simulink model "DynamicKviMultiMicrogrid"  (R2022b)
settings: Solver=ode45  StartTime=0.0  StopTime=1000  RelTol=1e-3
values from neighbouring files (symbols this model uses):
  a_hidden_weights1 = zeros(n,h)    [Weights.m]
  a_hidden_weights2 = zeros(n,h)    [Weights.m]
  a_hidden_weights3 = zeros(n,h)    [Weights.m]
  a_input_weights1 = zeros(h,m)    [Weights.m]
  a_input_weights2 = zeros(h,m)    [Weights.m]
  a_input_weights3 = zeros(h,m)    [Weights.m]
  c_hidden_weights11 = zeros(100,1000)    [Training.m]
  c_hidden_weights12 = -1+(1+1)*rand(1,100,'single')    [Training.m]
  c_hidden_weights21 = zeros(100,1000)    [Training.m]
  c_hidden_weights22 = -1+(1+1)*rand(1,100,'single')    [Training.m]
  c_hidden_weights31 = zeros(100,1000)    [Training.m]
  c_hidden_weights32 = -1+(1+1)*rand(1,100,'single')    [Training.m]
  c_hidden_weights_a1 = -1+(1+1)*rand(1,100,'single')    [Training.m]
  c_hidden_weights_a2 = -1+(1+1)*rand(1,100,'single')    [Training.m]
  c_hidden_weights_a3 = -1+(1+1)*rand(1,100,'single')    [Training.m]
  c_input_weights1 = zeros(1000,m)    [Training.m]
  c_input_weights2 = zeros(1000,m)    [Training.m]
  c_input_weights3 = zeros(1000,m)    [Training.m]
  c_input_weights_a1 = zeros(100,n)    [Training.m]
  c_input_weights_a2 = zeros(100,n)    [Training.m]
  c_input_weights_a3 = zeros(100,n)    [Training.m]
libraries: simulink x9, slpidlib x3
settings Model: Creator=Vjatšeslav Škiparev  LastModifiedBy=assned
settings DataIOCC: LoggingIntervals=[0, 1000]
settings DebuggingCC: UnconnectedInputMsg=warning  UnconnectedOutputMsg=warning  UnconnectedLineMsg=warning
settings HardwareCC: ProdBitPerLong=64  ProdHWDeviceType=Intel->x86-64 (Linux 64)
settings ModelReferenceCC: EnableRefExpFcnMdlSchedulingChecks=on
settings RTWCC: DLArmComputeVersion=19.05

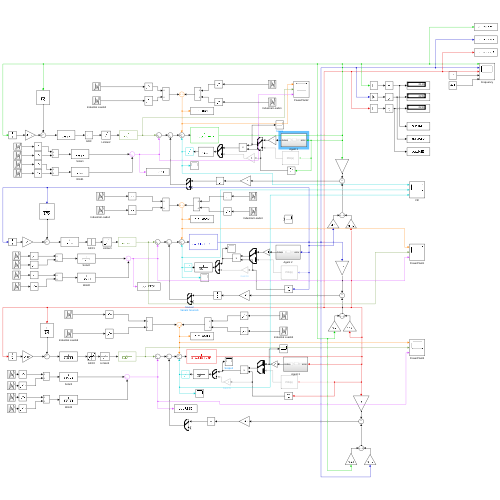
[thumbnail: Simulink's stored preview of the top-level diagram]
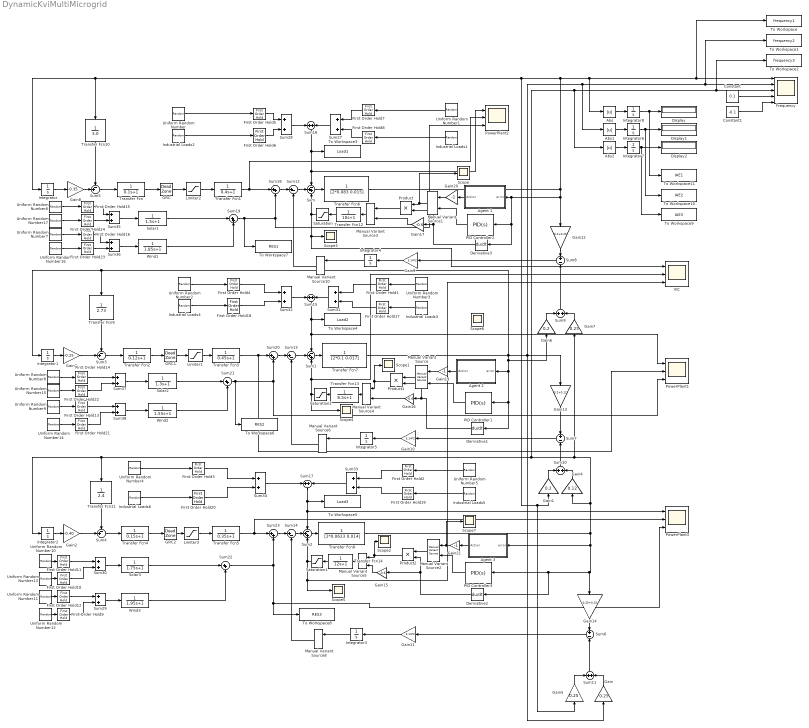
== system DynamicKviMultiMicrogrid ==
  Abs : Abs  SaturateOnIntegerOverflow=off
  Abs1 : Abs  SaturateOnIntegerOverflow=off
  Abs2 : Abs  SaturateOnIntegerOverflow=off
  Agent 1 : Subsystem
  Agent 2 : Subsystem
  Agent 3 : Subsystem
  Constant : Constant  Value=0.1
  Constant1 : Constant  Value=-0.1
  Derivative1 : Derivative
  Derivative2 : Derivative
  Derivative3 : Derivative
  Display : Display
  Display1 : Display
  Display2 : Display
  First Order Hold{1..24} (24 alike) : FirstOrderHold  ErrorTolerance=inf
  Frequency : Scope  NumInputPorts=5
  GRC : DeadZone  LowerValue=-0.12  UpperValue=0.12
  GRC1 : DeadZone  LowerValue=-0.12  UpperValue=0.12
  GRC2 : DeadZone  LowerValue=-0.12  UpperValue=0.12
  Gain : Gain  Gain=0.25
  Gain1 : Gain  Gain=0.2
  Gain10 : Gain  Gain=3.14*2
  Gain11 : Gain  Gain=3.14*2
  Gain12 : Gain  Gain=0.2+0.25
  Gain13 : Gain  Gain=0.2+0.12
  Gain14 : Gain  Gain=0.25+0.25
  Gain15 : Gain  Gain=-0.6
  Gain16 : Gain  Gain=-0.6
  Gain17 : Gain  Gain=-0.6
  Gain19 : Gain  Gain=-1
  Gain2 : Gain  Gain=-0.40
  Gain20 : Gain  Gain=-1
  Gain21 : Gain  Gain=-1
  Gain3 : Gain  Gain=-0.25
  Gain4 : Gain  Gain=0.12
  Gain5 : Gain  Gain=0.25
  Gain6 : Gain  Gain=0.2
  Gain7 : Gain  Gain=0.25
  Gain8 : Gain  Gain=-0.35
  Gain9 : Gain  Gain=3.14*2
  Industrial Loads1 : UniformRandomNumber  Minimum=-0.01  Maximum=0.01  SampleTime=1
  Industrial Loads2 : UniformRandomNumber  Minimum=-0.05  Maximum=0.05  SampleTime=2
  Industrial Loads3 : UniformRandomNumber  Minimum=-0.03  Maximum=0.03  SampleTime=5
  Industrial Loads4 : UniformRandomNumber  Minimum=-0.03  Maximum=0.03  SampleTime=5
  Industrial Loads5 : UniformRandomNumber  Minimum=-0.01  Maximum=0.01  SampleTime=2
  Industrial Loads6 : UniformRandomNumber  Minimum=-0.01  Maximum=0.01  SampleTime=2
  Integrator{,1..8} (9 alike) : Integrator
  Limiter1 : Saturate  UpperLimit=0.4  LowerLimit=0
  Limiter2 : Saturate  LowerLimit=0
  Limiter3 : Saturate  UpperLimit=0.3  LowerLimit=0
  Manual Variant Source{,1..6,8,10} (9 alike) : simulink/Signal Routing/Manual Variant Source  NumChoices=2  LabelModeActiveChoice=V_1
  PID Controller1 : slpidlib/PID Controller  Controller=PID  Form=Parallel  TimeDomain=Continuous-time  UseExternalTs=off  SampleTime=-1  IntegratorMethod=Forward Euler  FilterMethod=Forward Euler  ControllerParametersSource=internal  P=7.5  I=0.75  UseKiTs=off  D=0  N=100  UseFilter=on  TunerSelectOption=Transfer Function Based (PID Tuner App)  InitialConditionSource=internal  InitialConditionForIntegrator=0  InitialConditionForFilter=0  DifferentiatorICPrevScaledInput=0  ExternalReset=none  TrackingMode=off  Kt=1  LimitOutput=off  SatLimitsSource=internal  UpperSaturationLimit=inf  LowerSaturationLimit=-inf  LinearizeAsGain=on  AntiWindupMode=none  Kb=1  LimitIntegrator=off  UpperIntegratorSaturationLimit=inf  LowerIntegratorSaturationLimit=-inf  POutMin=[]  POutMax=[]  IOutMin=[]  IOutMax=[]  DOutMin=[]  DOutMax=[]  NOutMin=[]  NOutMax=[]  SumOutMin=[]  SumOutMax=[]  SaturationOutMin=[]  SaturationOutMax=[]  PParamMin=[]  PParamMax=[]  IParamMin=[]  IParamMax=[]  DParamMin=[]  DParamMax=[]  NParamMin=[]  NParamMax=[]  KbParamMin=[]  KbParamMax=[]  KtParamMin=[]  KtParamMax=[]  KbOutMin=[]  KbOutMax=[]  KtOutMin=[]  KtOutMax=[]  IntegratorOutMin=[]  IntegratorOutMax=[]  FilterOutMin=[]  FilterOutMax=[]  SumI1OutMin=[]  SumI1OutMax=[]  SumI2OutMin=[]  SumI2OutMax=[]  SumI3OutMin=[]  SumI3OutMax=[]  SumI4OutMin=[]  SumI4OutMax=[]  SumDOutMin=[]  SumDOutMax=[]  DifferentiatorOutMin=[]  DifferentiatorOutMax=[]  FilterDiffOutCoefMin=[]  FilterDiffOutCoefMax=[]  ReciprocalOutMin=[]  ReciprocalOutMax=[]  SumDenOutMin=[]  SumDenOutMax=[]  SumNumOutMin=[]  SumNumOutMax=[]  DivideOutMin=[]  DivideOutMax=[]  UdiffTsProdOutMin=[]  UdiffTsProdOutMax=[]  NTsProdOutMin=[]  NTsProdOutMax=[]  UintegralTsProdOutMin=[]  UintegralTsProdOutMax=[]  UngainTsProdOutMin=[]  UngainTsProdOutMax=[]  ClampingZeroOutDataTypeStr=Inherit: Inherit via back propagation  ClampingZeroOutMin=[]  ClampingZeroOutMax=[]  FilterDenConstantOutDataTypeStr=Inherit: Inherit via back propagation  FilterDenConstantOutMin=[]  FilterDenConstantOutMax=[]  PCopyOutDataTypeStr=Inherit: Inherit via back propagation  PCopyOutMin=[]  PCopyOutMax=[]  NCopyOutDataTypeStr=Inherit: Inherit via back propagation  NCopyOutMin=[]  NCopyOutMax=[]  IntegratorContinuousStateAttributes=''  IntegratorStateMustResolveToSignalObject=off  IntegratorRTWStateStorageClass=Auto  FilterContinuousStateAttributes=''  FilterStateMustResolveToSignalObject=off  FilterRTWStateStorageClass=Auto  ParallelPVariant=InternalParameters  IdealPVariant=Disabled  IVariant=InternalParameters  DVariant=InternalParameters  IntegratorVariant=Continuous  SatVariant=Disabled  AWVariant=Passthrough  PCopyVariant=Disabled  TRVariant=Disabled  FdbkBlocksVariant=Forward  IdealPFdbkVariant=Disabled  SatFdbkVariant=Disabled  DerivativeFilterVariant=ContFilter  NVariant=InternalParameters  NCopyVariant=Disabled  FilterICVariant=InternalICsFilter  IntegratorICVariant=InternalICs  ExternalResetVariant=Disabled  TRSumVariant=Passthrough  SumFdbkVariant=Disabled  SumVariant=Sum_PID  TsampFilterVariant=InternalTs  TsampNgainVariant=Passthrough  TsampIntegralVariant=Passthrough  ExternalSaturationOutDataTypeStr=Inherit: Same as second input
  PID Controller2 : slpidlib/PID Controller  Controller=PID  Form=Parallel  TimeDomain=Continuous-time  UseExternalTs=off  SampleTime=-1  IntegratorMethod=Forward Euler  FilterMethod=Forward Euler  ControllerParametersSource=internal  P=3.5  I=0.25  UseKiTs=off  D=0.5  N=100  UseFilter=on  TunerSelectOption=Transfer Function Based (PID Tuner App)  InitialConditionSource=internal  InitialConditionForIntegrator=0  InitialConditionForFilter=0  DifferentiatorICPrevScaledInput=0  ExternalReset=none  TrackingMode=off  Kt=1  LimitOutput=off  SatLimitsSource=internal  UpperSaturationLimit=inf  LowerSaturationLimit=-inf  LinearizeAsGain=on  AntiWindupMode=none  Kb=1  LimitIntegrator=off  UpperIntegratorSaturationLimit=inf  LowerIntegratorSaturationLimit=-inf  POutMin=[]  POutMax=[]  IOutMin=[]  IOutMax=[]  DOutMin=[]  DOutMax=[]  NOutMin=[]  NOutMax=[]  SumOutMin=[]  SumOutMax=[]  SaturationOutMin=[]  SaturationOutMax=[]  PParamMin=[]  PParamMax=[]  IParamMin=[]  IParamMax=[]  DParamMin=[]  DParamMax=[]  NParamMin=[]  NParamMax=[]  KbParamMin=[]  KbParamMax=[]  KtParamMin=[]  KtParamMax=[]  KbOutMin=[]  KbOutMax=[]  KtOutMin=[]  KtOutMax=[]  IntegratorOutMin=[]  IntegratorOutMax=[]  FilterOutMin=[]  FilterOutMax=[]  SumI1OutMin=[]  SumI1OutMax=[]  SumI2OutMin=[]  SumI2OutMax=[]  SumI3OutMin=[]  SumI3OutMax=[]  SumI4OutMin=[]  SumI4OutMax=[]  SumDOutMin=[]  SumDOutMax=[]  DifferentiatorOutMin=[]  DifferentiatorOutMax=[]  FilterDiffOutCoefMin=[]  FilterDiffOutCoefMax=[]  ReciprocalOutMin=[]  ReciprocalOutMax=[]  SumDenOutMin=[]  SumDenOutMax=[]  SumNumOutMin=[]  SumNumOutMax=[]  DivideOutMin=[]  DivideOutMax=[]  UdiffTsProdOutMin=[]  UdiffTsProdOutMax=[]  NTsProdOutMin=[]  NTsProdOutMax=[]  UintegralTsProdOutMin=[]  UintegralTsProdOutMax=[]  UngainTsProdOutMin=[]  UngainTsProdOutMax=[]  ClampingZeroOutDataTypeStr=Inherit: Inherit via back propagation  ClampingZeroOutMin=[]  ClampingZeroOutMax=[]  FilterDenConstantOutDataTypeStr=Inherit: Inherit via back propagation  FilterDenConstantOutMin=[]  FilterDenConstantOutMax=[]  PCopyOutDataTypeStr=Inherit: Inherit via back propagation  PCopyOutMin=[]  PCopyOutMax=[]  NCopyOutDataTypeStr=Inherit: Inherit via back propagation  NCopyOutMin=[]  NCopyOutMax=[]  IntegratorContinuousStateAttributes=''  IntegratorStateMustResolveToSignalObject=off  IntegratorRTWStateStorageClass=Auto  FilterContinuousStateAttributes=''  FilterStateMustResolveToSignalObject=off  FilterRTWStateStorageClass=Auto  ParallelPVariant=InternalParameters  IdealPVariant=Disabled  IVariant=InternalParameters  DVariant=InternalParameters  IntegratorVariant=Continuous  SatVariant=Disabled  AWVariant=Passthrough  PCopyVariant=Disabled  TRVariant=Disabled  FdbkBlocksVariant=Forward  IdealPFdbkVariant=Disabled  SatFdbkVariant=Disabled  DerivativeFilterVariant=ContFilter  NVariant=InternalParameters  NCopyVariant=Disabled  FilterICVariant=InternalICsFilter  IntegratorICVariant=InternalICs  ExternalResetVariant=Disabled  TRSumVariant=Passthrough  SumFdbkVariant=Disabled  SumVariant=Sum_PID  TsampFilterVariant=InternalTs  TsampNgainVariant=Passthrough  TsampIntegralVariant=Passthrough  ExternalSaturationOutDataTypeStr=Inherit: Same as second input
  PID Controller3 : slpidlib/PID Controller  Controller=PID  Form=Parallel  TimeDomain=Continuous-time  UseExternalTs=off  SampleTime=-1  IntegratorMethod=Forward Euler  FilterMethod=Forward Euler  ControllerParametersSource=internal  P=7.5  I=0.05  UseKiTs=off  D=0  N=100  UseFilter=on  TunerSelectOption=Transfer Function Based (PID Tuner App)  InitialConditionSource=internal  InitialConditionForIntegrator=0  InitialConditionForFilter=0  DifferentiatorICPrevScaledInput=0  ExternalReset=none  TrackingMode=off  Kt=1  LimitOutput=off  SatLimitsSource=internal  UpperSaturationLimit=inf  LowerSaturationLimit=-inf  LinearizeAsGain=on  AntiWindupMode=none  Kb=1  LimitIntegrator=off  UpperIntegratorSaturationLimit=inf  LowerIntegratorSaturationLimit=-inf  POutMin=[]  POutMax=[]  IOutMin=[]  IOutMax=[]  DOutMin=[]  DOutMax=[]  NOutMin=[]  NOutMax=[]  SumOutMin=[]  SumOutMax=[]  SaturationOutMin=[]  SaturationOutMax=[]  PParamMin=[]  PParamMax=[]  IParamMin=[]  IParamMax=[]  DParamMin=[]  DParamMax=[]  NParamMin=[]  NParamMax=[]  KbParamMin=[]  KbParamMax=[]  KtParamMin=[]  KtParamMax=[]  KbOutMin=[]  KbOutMax=[]  KtOutMin=[]  KtOutMax=[]  IntegratorOutMin=[]  IntegratorOutMax=[]  FilterOutMin=[]  FilterOutMax=[]  SumI1OutMin=[]  SumI1OutMax=[]  SumI2OutMin=[]  SumI2OutMax=[]  SumI3OutMin=[]  SumI3OutMax=[]  SumI4OutMin=[]  SumI4OutMax=[]  SumDOutMin=[]  SumDOutMax=[]  DifferentiatorOutMin=[]  DifferentiatorOutMax=[]  FilterDiffOutCoefMin=[]  FilterDiffOutCoefMax=[]  ReciprocalOutMin=[]  ReciprocalOutMax=[]  SumDenOutMin=[]  SumDenOutMax=[]  SumNumOutMin=[]  SumNumOutMax=[]  DivideOutMin=[]  DivideOutMax=[]  UdiffTsProdOutMin=[]  UdiffTsProdOutMax=[]  NTsProdOutMin=[]  NTsProdOutMax=[]  UintegralTsProdOutMin=[]  UintegralTsProdOutMax=[]  UngainTsProdOutMin=[]  UngainTsProdOutMax=[]  ClampingZeroOutDataTypeStr=Inherit: Inherit via back propagation  ClampingZeroOutMin=[]  ClampingZeroOutMax=[]  FilterDenConstantOutDataTypeStr=Inherit: Inherit via back propagation  FilterDenConstantOutMin=[]  FilterDenConstantOutMax=[]  PCopyOutDataTypeStr=Inherit: Inherit via back propagation  PCopyOutMin=[]  PCopyOutMax=[]  NCopyOutDataTypeStr=Inherit: Inherit via back propagation  NCopyOutMin=[]  NCopyOutMax=[]  IntegratorContinuousStateAttributes=''  IntegratorStateMustResolveToSignalObject=off  IntegratorRTWStateStorageClass=Auto  FilterContinuousStateAttributes=''  FilterStateMustResolveToSignalObject=off  FilterRTWStateStorageClass=Auto  ParallelPVariant=InternalParameters  IdealPVariant=Disabled  IVariant=InternalParameters  DVariant=InternalParameters  IntegratorVariant=Continuous  SatVariant=Disabled  AWVariant=Passthrough  PCopyVariant=Disabled  TRVariant=Disabled  FdbkBlocksVariant=Forward  IdealPFdbkVariant=Disabled  SatFdbkVariant=Disabled  DerivativeFilterVariant=ContFilter  NVariant=InternalParameters  NCopyVariant=Disabled  FilterICVariant=InternalICsFilter  IntegratorICVariant=InternalICs  ExternalResetVariant=Disabled  TRSumVariant=Passthrough  SumFdbkVariant=Disabled  SumVariant=Sum_PID  TsampFilterVariant=InternalTs  TsampNgainVariant=Passthrough  TsampIntegralVariant=Passthrough  ExternalSaturationOutDataTypeStr=Inherit: Same as second input
  PowerPlant1 : Scope  NumInputPorts=3
  PowerPlant2 : Scope  NumInputPorts=3
  PowerPlant3 : Scope  NumInputPorts=3
  Product : Product
  Product1 : Product
  Product2 : Product
  Saturation : Saturate  UpperLimit=0.25  LowerLimit=-0.25
  Saturation1 : Saturate  UpperLimit=0.1  LowerLimit=-0.1
  Saturation2 : Saturate  UpperLimit=0.25  LowerLimit=-0.25
  Scope{,1..7} (8 alike) : Scope
  Solar1 : TransferFcn  Denominator=[1.5 1]
  Solar2 : TransferFcn  Denominator=[1.3 1]
  Solar3 : TransferFcn  Denominator=[1.75 1]
  Sum : Sum  Inputs=-++
  Sum1 : Sum  Inputs=-++
  Sum{9..11,15..17,27..38} (18 alike) : Sum
  Sum12 : Sum  Inputs=|+-
  Sum13 : Sum  Inputs=|+-
  Sum14 : Sum  Inputs=|+-
  Sum{18..23} (6 alike) : Sum  Inputs=|++
  Sum2 : Sum  Inputs=-++
  Sum3 : Sum  Inputs=-+|
  Sum4 : Sum  Inputs=-+|
  Sum5 : Sum  Inputs=-+|
  Sum6 : Sum  Inputs=+-
  Sum7 : Sum  Inputs=+-
  Sum8 : Sum  Inputs=+-
  To Workspace : ToWorkspace  VariableName=frequency1  SampleTime=1
  To Workspace1 : ToWorkspace  VariableName=frequency2  SampleTime=1
  To Workspace10 : ToWorkspace  VariableName=IAE2  SampleTime=1
  To Workspace11 : ToWorkspace  VariableName=IAE1  SampleTime=1
  To Workspace2 : ToWorkspace  VariableName=frequency3  SampleTime=1
  To Workspace3 : ToWorkspace  VariableName=Load1  SampleTime=1
  To Workspace4 : ToWorkspace  VariableName=Load2  SampleTime=1
  To Workspace5 : ToWorkspace  VariableName=Load3  SampleTime=1
  To Workspace6 : ToWorkspace  VariableName=RES2  SampleTime=1
  To Workspace7 : ToWorkspace  VariableName=RES1  SampleTime=1
  To Workspace8 : ToWorkspace  VariableName=RES3  SampleTime=1
  To Workspace9 : ToWorkspace  VariableName=IAE3  SampleTime=1
  Transfer Fcn : TransferFcn  Denominator=[0.1 1]
  Transfer Fcn1 : TransferFcn  Denominator=[0.4 1]
  Transfer Fcn10 : TransferFcn  Denominator=[3.0]
  Transfer Fcn11 : TransferFcn  Denominator=[2.4]
  Transfer Fcn12 : TransferFcn  Denominator=[10 1]
  Transfer Fcn13 : TransferFcn  Denominator=[8.5 1]
  Transfer Fcn14 : TransferFcn  Denominator=[12 1]
  Transfer Fcn2 : TransferFcn  Denominator=[0.12 1]
  Transfer Fcn3 : TransferFcn  Denominator=[0.45 1]
  Transfer Fcn4 : TransferFcn  Denominator=[0.15 1]
  Transfer Fcn5 : TransferFcn  Denominator=[0.35 1]
  Transfer Fcn6 : TransferFcn  Denominator=[2*0.083 0.015]
  Transfer Fcn7 : TransferFcn  Denominator=[2*0.1 0.017]
  Transfer Fcn8 : TransferFcn  Denominator=[2*0.0623 0.014]
  Transfer Fcn9 : TransferFcn  Denominator=[2.73]
  Uniform Random Number : UniformRandomNumber  Minimum=0.15  Maximum=0.25  SampleTime=25
  Uniform Random Number1 : UniformRandomNumber  Minimum=0.35  Maximum=0.40  SampleTime=25
  Uniform Random Number10 : UniformRandomNumber  Minimum=0.05  Maximum=0.075  SampleTime=10
  Uniform Random Number11 : UniformRandomNumber  Minimum=0.05  Maximum=0.075  SampleTime=10
  Uniform Random Number12 : UniformRandomNumber  Minimum=-0.01  Maximum=0.01  SampleTime=1
  Uniform Random Number13 : UniformRandomNumber  Minimum=-0.05  Maximum=0.05  SampleTime=1
  Uniform Random Number14 : UniformRandomNumber  Minimum=-0.01  Maximum=0.01  SampleTime=1
  Uniform Random Number15 : UniformRandomNumber  Minimum=-0.01  Maximum=0.01  SampleTime=1
  Uniform Random Number16 : UniformRandomNumber  Minimum=-0.015  Maximum=0.015  SampleTime=2
  Uniform Random Number17 : UniformRandomNumber  Minimum=-0.015  Maximum=0.015  SampleTime=2
  Uniform Random Number2 : UniformRandomNumber  Minimum=0.2  Maximum=0.30  SampleTime=3
  Uniform Random Number3 : UniformRandomNumber  Minimum=0.225  Maximum=0.275  SampleTime=5
  Uniform Random Number4 : UniformRandomNumber  Minimum=0.15  Maximum=0.2  SampleTime=15
  Uniform Random Number5 : UniformRandomNumber  Minimum=0.075  Maximum=0.10  SampleTime=15
  Uniform Random Number6 : UniformRandomNumber  Minimum=0.10  Maximum=0.15  SampleTime=20
  Uniform Random Number7 : UniformRandomNumber  Minimum=0.10  Maximum=0.15  SampleTime=20
  Uniform Random Number8 : UniformRandomNumber  Minimum=0.125  Maximum=0.15  SampleTime=15
  Uniform Random Number9 : UniformRandomNumber  Minimum=0.05  Maximum=0.10  SampleTime=15
  VIC : Scope  NumInputPorts=3
  Wind1 : TransferFcn  Denominator=[1.85 1]
  Wind2 : TransferFcn  Denominator=[1.55 1]
  Wind3 : TransferFcn  Denominator=[1.95 1]
  wires:
  Sum1/1 -> Transfer Fcn7/1
  Sum2/1 -> Transfer Fcn8/1
  Sum/1 -> Transfer Fcn6/1
  Integrator/1 -> Gain8/1
  Sum5/1 -> Transfer Fcn/1
  Sum3/1 -> Transfer Fcn2/1
  Integrator1/1 -> Gain3/1
  Integrator2/1 -> Gain2/1
  Sum4/1 -> Transfer Fcn4/1
  Transfer Fcn9/1 -> Sum3/1
  Transfer Fcn10/1 -> Sum5/1
  Transfer Fcn11/1 -> Sum4/1
  Gain5/1 -> Sum11/1
  Gain/1 -> Sum11/2
  Gain4/1 -> Sum10/2
  Gain1/1 -> Sum10/1
  Gain3/1 -> Sum3/2
  Gain2/1 -> Sum4/2
  Gain6/1 -> Sum9/1
  Gain7/1 -> Sum9/2
  Gain8/1 -> Sum5/2
  Transfer Fcn14/1 -> Saturation1/1
  Saturation2/1 -> VIC/2, Sum1/3, Scope4/1
  Transfer Fcn12/1 -> Saturation/1
  Sum15/1 -> PowerPlant1/1, Sum1/1, To Workspace4/1
  Sum16/1 -> PowerPlant2/1, Sum/1, To Workspace3/1
  Sum17/1 -> To Workspace5/1, Sum2/1, PowerPlant3/1
  Uniform Random Number/1 -> First Order Hold5/1
  Uniform Random Number1/1 -> First Order Hold7/1
  Uniform Random Number2/1 -> First Order Hold4/1
  Uniform Random Number3/1 -> First Order Hold1/1
  Uniform Random Number4/1 -> First Order Hold3/1
  Uniform Random Number5/1 -> First Order Hold2/1
  Uniform Random Number6/1 -> First Order Hold15/1
  Uniform Random Number7/1 -> First Order Hold16/1
  Transfer Fcn1/1 -> Sum18/1, PowerPlant2/2
  Sum19/1 -> Sum18/2, PowerPlant2/3, To Workspace7/1
  Transfer Fcn3/1 -> PowerPlant1/2, Sum20/1
  Sum21/1 -> Sum20/2, PowerPlant1/3, To Workspace6/1
  Uniform Random Number8/1 -> First Order Hold14/1
  Uniform Random Number9/1 -> First Order Hold13/1
  Transfer Fcn5/1 -> PowerPlant3/2, Sum23/1
  Transfer Fcn13/1 -> Saturation2/1
  Saturation1/1 -> Sum2/3, Scope5/1, VIC/3
  Saturation/1 -> Sum/3, Scope3/1, VIC/1
  Wind3/1 -> Sum22/2
  Solar3/1 -> Sum22/1
  Solar2/1 -> Sum21/1
  Wind2/1 -> Sum21/2
  Wind1/1 -> Sum19/2
  Solar1/1 -> Sum19/1
  GRC/1 -> Limiter2/1
  Transfer Fcn/1 -> GRC/1
  Limiter2/1 -> Transfer Fcn1/1
  GRC1/1 -> Limiter1/1
  Transfer Fcn2/1 -> GRC1/1
  Limiter1/1 -> Transfer Fcn3/1
  GRC2/1 -> Limiter3/1
  Limiter3/1 -> Transfer Fcn5/1
  Transfer Fcn4/1 -> GRC2/1
  Sum18/1 -> Sum12/1
  Sum12/1 -> Sum/2
  Sum20/1 -> Sum13/1
  Sum13/1 -> Sum1/2
  Sum23/1 -> Sum14/1
  Sum14/1 -> Sum2/2
  Transfer Fcn6/1 -> Gain12/1, Derivative3/1, PID Controller2/1, Agent 1/1(error), Integrator/1, Transfer Fcn10/1, Gain1/1, Gain5/1, Abs/1, Frequency/1, To Workspace/1
  Sum8/1 -> Gain9/1
  Sum7/1 -> Gain10/1
  Sum6/1 -> Gain11/1
  First Order Hold7/1 -> Sum27/1
  Sum27/1 -> Sum16/2
  First Order Hold8/1 -> Sum27/2
  Industrial Loads1/1 -> First Order Hold8/1
  Sum28/1 -> Sum16/1
  First Order Hold5/1 -> Sum28/1
  First Order Hold6/1 -> Sum28/2
  Industrial Loads2/1 -> First Order Hold6/1
  First Order Hold9/1 -> Sum29/2
  Uniform Random Number12/1 -> First Order Hold9/1
  Uniform Random Number11/1 -> First Order Hold12/1
  Sum29/1 -> Wind3/1
  Uniform Random Number10/1 -> First Order Hold11/1
  Sum30/1 -> Solar3/1
  First Order Hold10/1 -> Sum30/2
  Uniform Random Number13/1 -> First Order Hold10/1
  First Order Hold11/1 -> Sum30/1
  First Order Hold12/1 -> Sum29/1
  First Order Hold17/1 -> Sum31/2
  Industrial Loads3/1 -> First Order Hold17/1
  First Order Hold1/1 -> Sum31/1
  Industrial Loads4/1 -> First Order Hold18/1
  First Order Hold18/1 -> Sum32/2
  First Order Hold4/1 -> Sum32/1
  Sum32/1 -> Sum15/1
  First Order Hold19/1 -> Sum33/2
  Industrial Loads5/1 -> First Order Hold19/1
  First Order Hold2/1 -> Sum33/1
  Sum33/1 -> Sum17/2
  First Order Hold20/1 -> Sum34/2
  Industrial Loads6/1 -> First Order Hold20/1
  Sum34/1 -> Sum17/1
  First Order Hold3/1 -> Sum34/1
  Manual Variant Source10/1 -> Sum12/2
  Manual Variant Source8/1 -> Sum14/2
  Manual Variant Source6/1 -> Sum13/2
  Gain9/1 -> Integrator4/1
  Gain10/1 -> Integrator5/1
  Gain11/1 -> Integrator3/1
  Gain12/1 -> Sum8/1
  Gain13/1 -> Sum7/1
  Gain14/1 -> Sum6/1
  PID Controller1/1 -> Manual Variant Source/2
  PID Controller3/1 -> Manual Variant Source2/2
  Sum35/1 -> Solar1/1
  First Order Hold15/1 -> Sum35/1
  Sum36/1 -> Wind1/1
  First Order Hold16/1 -> Sum36/1
  Sum37/1 -> Solar2/1
  Sum38/1 -> Wind2/1
  First Order Hold14/1 -> Sum37/1
  First Order Hold13/1 -> Sum38/1
  Uniform Random Number14/1 -> First Order Hold21/1
  First Order Hold21/1 -> Sum38/2
  Uniform Random Number15/1 -> First Order Hold22/1
  First Order Hold22/1 -> Sum37/2
  First Order Hold23/1 -> Sum36/2
  Uniform Random Number16/1 -> First Order Hold23/1
  Uniform Random Number17/1 -> First Order Hold24/1
  First Order Hold24/1 -> Sum35/2
  Integrator8/1 -> To Workspace11/1, Display/1
  Integrator6/1 -> To Workspace10/1, Display1/1
  Abs2/1 -> Integrator7/1
  Constant/1 -> Frequency/4
  Constant1/1 -> Frequency/5
  PID Controller2/1 -> Manual Variant Source1/2
  Manual Variant Source/1 -> Product1/1
  Manual Variant Source2/1 -> Product2/1
  Manual Variant Source4/1 -> Transfer Fcn13/1
  Manual Variant Source5/1 -> Transfer Fcn14/1
  Manual Variant Source3/1 -> Transfer Fcn12/1
  Gain16/1 -> Manual Variant Source4/2
  Gain17/1 -> Manual Variant Source3/2
  Derivative3/1 -> Gain17/1, Product/2
  Derivative1/1 -> Gain16/1, Product1/2
  Derivative2/1 -> Gain15/1, Product2/2
  Transfer Fcn7/1 -> Agent 2/1(error), PID Controller1/1, Derivative1/1, Gain6/1, Integrator1/1, Transfer Fcn9/1, Gain13/1, Gain/1, Abs1/1, To Workspace1/1, Frequency/2
  Product/1 -> Manual Variant Source3/1
  Product1/1 -> Scope1/1, Manual Variant Source4/1
  Product2/1 -> Scope2/1, Manual Variant Source5/1
  Gain15/1 -> Manual Variant Source5/2
  Sum9/1 -> Sum8/2
  Sum10/1 -> Sum7/2
  Sum11/1 -> Sum6/2
  Sum31/1 -> Sum15/2
  Abs/1 -> Integrator8/1
  Integrator7/1 -> Display2/1, To Workspace9/1
  Abs1/1 -> Integrator6/1
  Integrator5/1 -> Manual Variant Source6/1
  Integrator3/1 -> Manual Variant Source8/1
  Integrator4/1 -> Manual Variant Source10/1
  Transfer Fcn8/1 -> Integrator2/1, Transfer Fcn11/1, To Workspace2/1, Frequency/3, Abs2/1, Gain7/1, Gain4/1, Derivative2/1, PID Controller3/1, Gain14/1, Agent 3/1(error)
  Sum22/1 -> PowerPlant3/3, To Workspace8/1, Sum23/2
  Manual Variant Source1/1 -> Scope/1, Product/1
  Gain20/1 -> Manual Variant Source1/1
  Agent 1/1(Action) -> Gain20/1
  Gain19/1 -> Manual Variant Source/1
  Agent 2/1(Action) -> Gain19/1
  Gain21/1 -> Scope7/1, Manual Variant Source2/1
  Agent 3/1(Action) -> Gain21/1

== system DynamicKviMultiMicrogrid/Agent 1 ==
  error : Inport
  Gamma : Subsystem
  generate observations : Subsystem
  Action : Outport
  wires:
  error/1 -> Gamma/2(error), generate observations/1(error)
  generate observations/1(observations) -> Gamma/1(observations)
  Gamma/1(Action) -> Action/1

== system DynamicKviMultiMicrogrid/Agent 2 ==
  error : Inport
  Gamma : Subsystem
  generate observations : Subsystem
  Action : Outport
  wires:
  error/1 -> Gamma/2(error), generate observations/1(error)
  generate observations/1(observations) -> Gamma/1(observations)
  Gamma/1(Action) -> Action/1

== system DynamicKviMultiMicrogrid/Agent 3 ==
  error : Inport
  Gamma : Subsystem
  generate observations : Subsystem
  Action : Outport
  wires:
  error/1 -> Gamma/2(error), generate observations/1(error)
  generate observations/1(observations) -> Gamma/1(observations)
  Gamma/1(Action) -> Action/1

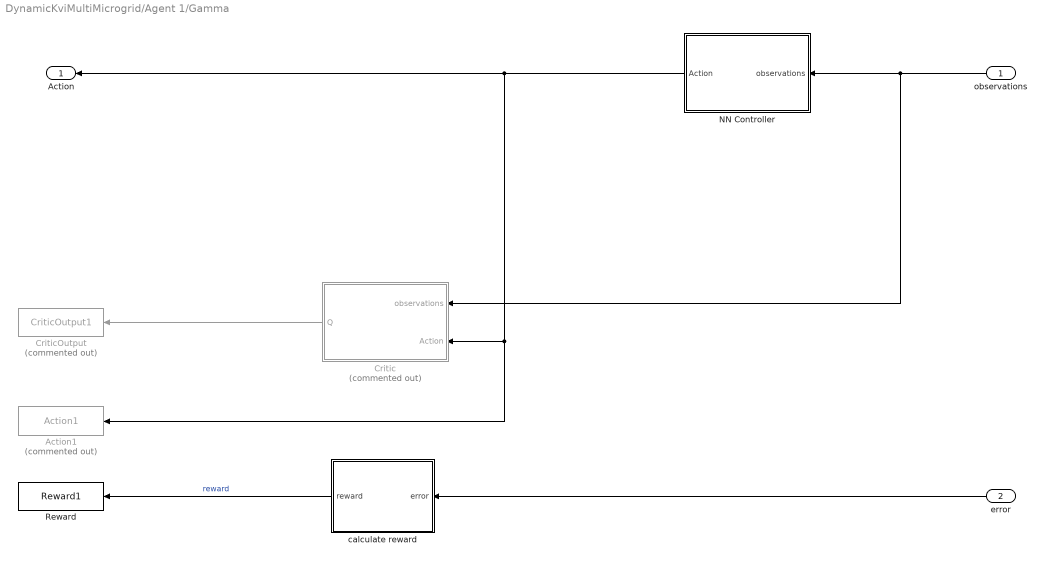
== system DynamicKviMultiMicrogrid/Agent 1/Gamma ==
  observations : Inport
  error : Inport  Port=2
  Action1 : ToWorkspace  Commented=on  VariableName=Action1  SampleTime=1
      settings: Save2DSignal=2-D array (concatenate along first dimension)
  Critic : Subsystem  Commented=on
  CriticOutput : ToWorkspace  Commented=on  VariableName=CriticOutput1  SampleTime=1
      settings: Save2DSignal=2-D array (concatenate along first dimension)
  NN Controller : Subsystem
  Reward : ToWorkspace  VariableName=Reward1  SampleTime=1
      settings: Save2DSignal=2-D array (concatenate along first dimension)
  calculate reward : Subsystem
  Action : Outport
  wires:
  NN Controller/1(Action) -> Action1/1, Critic/2(Action), Action/1
  observations/1 -> Critic/1(observations), NN Controller/1(observations)
  calculate reward/1(reward) -> Reward/1  "reward"
  Critic/1(Q) -> CriticOutput/1
  error/1 -> calculate reward/1(error)

== system DynamicKviMultiMicrogrid/Agent 1/generate observations ==
  error : Inport
  Derivative : Derivative
  Integrator : Integrator  IgnoreLimit=on
  Mux : Mux  Inputs=3
  observations : Outport  VectorParamsAs1DForOutWhenUnconnected=off
  wires:
  Mux/1 -> observations/1
  Integrator/1 -> Mux/2
  Derivative/1 -> Mux/3
  error/1 -> Derivative/1, Mux/1, Integrator/1

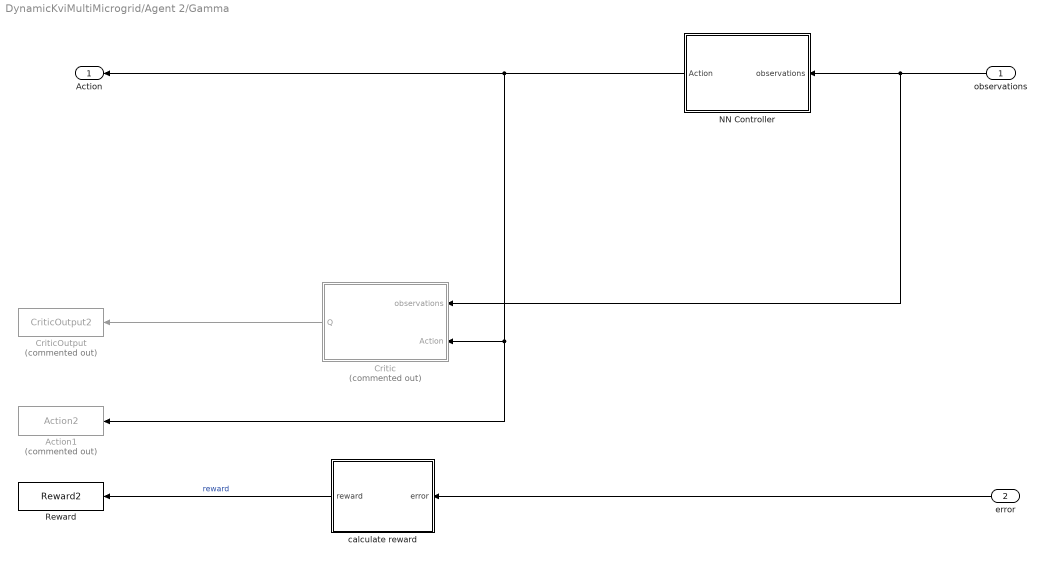
== system DynamicKviMultiMicrogrid/Agent 2/Gamma ==
  observations : Inport
  error : Inport  Port=2
  Action1 : ToWorkspace  Commented=on  VariableName=Action2  SampleTime=1
      settings: Save2DSignal=2-D array (concatenate along first dimension)
  Critic : Subsystem  Commented=on
  CriticOutput : ToWorkspace  Commented=on  VariableName=CriticOutput2  SampleTime=1
      settings: Save2DSignal=2-D array (concatenate along first dimension)
  NN Controller : Subsystem
  Reward : ToWorkspace  VariableName=Reward2  SampleTime=1
      settings: Save2DSignal=2-D array (concatenate along first dimension)
  calculate reward : Subsystem
  Action : Outport
  wires:
  NN Controller/1(Action) -> Action1/1, Critic/2(Action), Action/1
  observations/1 -> Critic/1(observations), NN Controller/1(observations)
  calculate reward/1(reward) -> Reward/1  "reward"
  Critic/1(Q) -> CriticOutput/1
  error/1 -> calculate reward/1(error)

== system DynamicKviMultiMicrogrid/Agent 2/generate observations ==
  error : Inport
  Derivative : Derivative
  Integrator : Integrator  IgnoreLimit=on
  Mux : Mux  Inputs=3
  observations : Outport  VectorParamsAs1DForOutWhenUnconnected=off
  wires:
  Mux/1 -> observations/1
  error/1 -> Derivative/1, Integrator/1, Mux/1
  Integrator/1 -> Mux/2
  Derivative/1 -> Mux/3

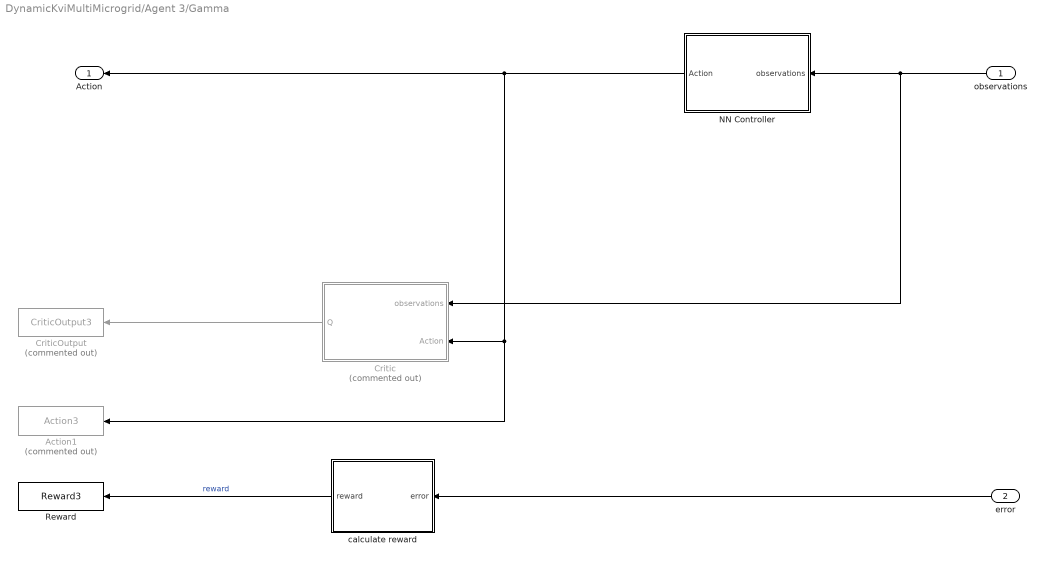
== system DynamicKviMultiMicrogrid/Agent 3/Gamma ==
  observations : Inport
  error : Inport  Port=2
  Action1 : ToWorkspace  Commented=on  VariableName=Action3  SampleTime=1
      settings: Save2DSignal=2-D array (concatenate along first dimension)
  Critic : Subsystem  Commented=on
  CriticOutput : ToWorkspace  Commented=on  VariableName=CriticOutput3  SampleTime=1
      settings: Save2DSignal=2-D array (concatenate along first dimension)
  NN Controller : Subsystem
  Reward : ToWorkspace  VariableName=Reward3  SampleTime=1
      settings: Save2DSignal=2-D array (concatenate along first dimension)
  calculate reward : Subsystem
  Action : Outport
  wires:
  NN Controller/1(Action) -> Action1/1, Critic/2(Action), Action/1
  observations/1 -> Critic/1(observations), NN Controller/1(observations)
  calculate reward/1(reward) -> Reward/1  "reward"
  Critic/1(Q) -> CriticOutput/1
  error/1 -> calculate reward/1(error)

== system DynamicKviMultiMicrogrid/Agent 3/generate observations ==
  error : Inport
  Derivative : Derivative
  Integrator : Integrator  IgnoreLimit=on
  Mux : Mux  Inputs=3
  observations : Outport  VectorParamsAs1DForOutWhenUnconnected=off
  wires:
  Mux/1 -> observations/1
  error/1 -> Derivative/1, Integrator/1, Mux/1
  Integrator/1 -> Mux/2
  Derivative/1 -> Mux/3

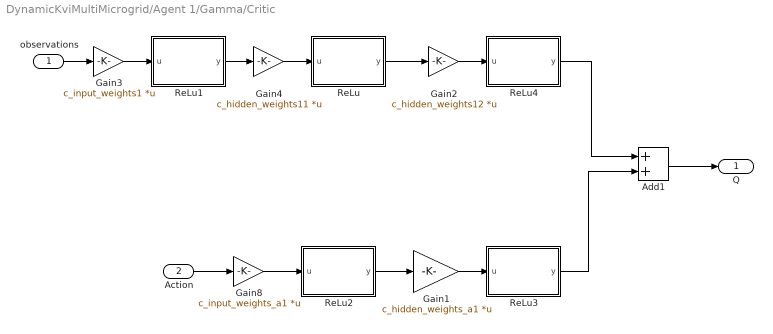
== system DynamicKviMultiMicrogrid/Agent 1/Gamma/Critic ==
  observations : Inport
  Action : Inport  Port=2
  Add1 : Sum
  Gain1 : Gain  Gain=c_hidden_weights_a1  Multiplication=Matrix(K*u)
  Gain2 : Gain  Gain=c_hidden_weights12  Multiplication=Matrix(K*u)
  Gain3 : Gain  Gain=c_input_weights1  Multiplication=Matrix(K*u)
  Gain4 : Gain  Gain=c_hidden_weights11  Multiplication=Matrix(K*u)
  Gain8 : Gain  Gain=c_input_weights_a1  Multiplication=Matrix(K*u)
  ReLu : MATLAB Function  TreatAsAtomicUnit=on
  ReLu1 : MATLAB Function  TreatAsAtomicUnit=on
  ReLu2 : MATLAB Function  TreatAsAtomicUnit=on
  ReLu3 : MATLAB Function  TreatAsAtomicUnit=on
  ReLu4 : MATLAB Function  TreatAsAtomicUnit=on
  Q : Outport
  wires:
  observations/1 -> Gain3/1
  Add1/1 -> Q/1
  Action/1 -> Gain8/1
  ReLu3/1(y) -> Add1/2
  Gain8/1 -> ReLu2/1(u)
  ReLu2/1(y) -> Gain1/1
  Gain1/1 -> ReLu3/1(u)
  Gain3/1 -> ReLu1/1(u)
  ReLu1/1(y) -> Gain4/1
  Gain4/1 -> ReLu/1(u)
  ReLu/1(y) -> Gain2/1
  Gain2/1 -> ReLu4/1(u)
  ReLu4/1(y) -> Add1/1

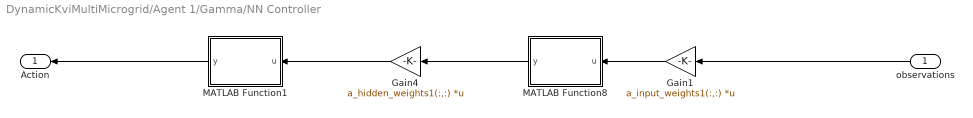
== system DynamicKviMultiMicrogrid/Agent 1/Gamma/NN Controller ==
  observations : Inport
  Gain1 : Gain  Gain=a_input_weights1(:,:)  Multiplication=Matrix(K*u)
  Gain4 : Gain  Gain=a_hidden_weights1(:,:)  Multiplication=Matrix(K*u)
  MATLAB Function1 : MATLAB Function  TreatAsAtomicUnit=on
  MATLAB Function8 : MATLAB Function  TreatAsAtomicUnit=on
  Action : Outport
  wires:
  Gain1/1 -> MATLAB Function8/1(u)
  Gain4/1 -> MATLAB Function1/1(u)
  MATLAB Function8/1(y) -> Gain4/1
  observations/1 -> Gain1/1
  MATLAB Function1/1(y) -> Action/1

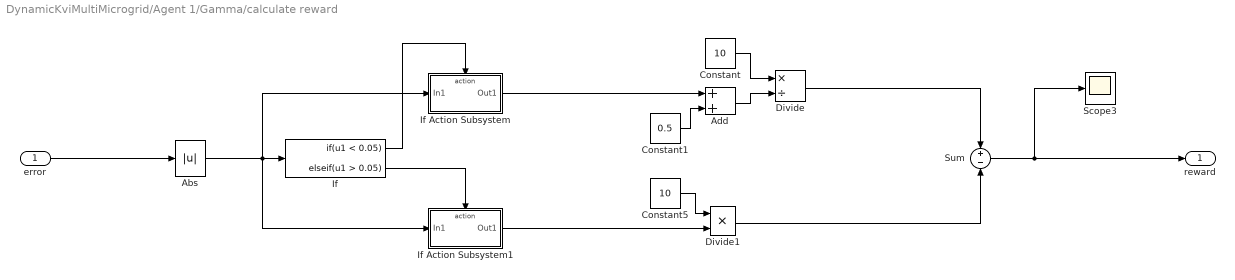
== system DynamicKviMultiMicrogrid/Agent 1/Gamma/calculate reward ==
  error : Inport
  Abs : Abs  SaturateOnIntegerOverflow=off
  Add : Sum
  Constant : Constant  Value=10
  Constant1 : Constant  Value=0.5  VectorParams1D=off
  Constant5 : Constant  Value=10  VectorParams1D=off
  Divide : Product  Inputs=*/
  Divide1 : Product  Inputs=**
  If : If  IfExpression=u1 < 0.05  ElseIfExpressions=u1 > 0.05  ShowElse=off
  If Action Subsystem : Subsystem  TreatAsAtomicUnit=on
  If Action Subsystem1 : Subsystem  TreatAsAtomicUnit=on
  Scope3 : Scope
  Sum : Sum  Inputs=+-  OutDataTypeStr=double
  reward : Outport  VectorParamsAs1DForOutWhenUnconnected=off
  wires:
  Constant/1 -> Divide/1
  Add/1 -> Divide/2
  Constant1/1 -> Add/2
  error/1 -> Abs/1
  Constant5/1 -> Divide1/1
  If Action Subsystem1/1(Out1) -> Divide1/2
  Divide/1 -> Sum/1
  If Action Subsystem/1(Out1) -> Add/1
  Sum/1 -> Scope3/1, reward/1
  If/2 -> If Action Subsystem1/Action
  If/1 -> If Action Subsystem/Action
  Abs/1 -> If/1, If Action Subsystem1/1(In1), If Action Subsystem/1(In1)
  Divide1/1 -> Sum/2

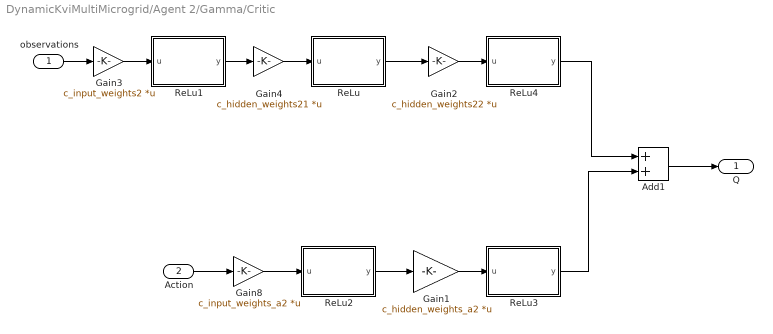
== system DynamicKviMultiMicrogrid/Agent 2/Gamma/Critic ==
  observations : Inport
  Action : Inport  Port=2
  Add1 : Sum
  Gain1 : Gain  Gain=c_hidden_weights_a2  Multiplication=Matrix(K*u)
  Gain2 : Gain  Gain=c_hidden_weights22  Multiplication=Matrix(K*u)
  Gain3 : Gain  Gain=c_input_weights2  Multiplication=Matrix(K*u)
  Gain4 : Gain  Gain=c_hidden_weights21  Multiplication=Matrix(K*u)
  Gain8 : Gain  Gain=c_input_weights_a2  Multiplication=Matrix(K*u)
  ReLu : MATLAB Function  TreatAsAtomicUnit=on
  ReLu1 : MATLAB Function  TreatAsAtomicUnit=on
  ReLu2 : MATLAB Function  TreatAsAtomicUnit=on
  ReLu3 : MATLAB Function  TreatAsAtomicUnit=on
  ReLu4 : MATLAB Function  TreatAsAtomicUnit=on
  Q : Outport
  wires:
  observations/1 -> Gain3/1
  Add1/1 -> Q/1
  Action/1 -> Gain8/1
  ReLu3/1(y) -> Add1/2
  Gain8/1 -> ReLu2/1(u)
  ReLu2/1(y) -> Gain1/1
  Gain1/1 -> ReLu3/1(u)
  Gain3/1 -> ReLu1/1(u)
  ReLu1/1(y) -> Gain4/1
  Gain4/1 -> ReLu/1(u)
  ReLu/1(y) -> Gain2/1
  Gain2/1 -> ReLu4/1(u)
  ReLu4/1(y) -> Add1/1

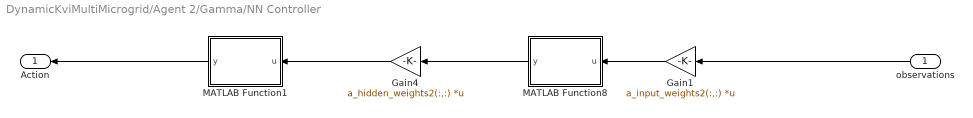
== system DynamicKviMultiMicrogrid/Agent 2/Gamma/NN Controller ==
  observations : Inport
  Gain1 : Gain  Gain=a_input_weights2(:,:)  Multiplication=Matrix(K*u)
  Gain4 : Gain  Gain=a_hidden_weights2(:,:)  Multiplication=Matrix(K*u)
  MATLAB Function1 : MATLAB Function  TreatAsAtomicUnit=on
  MATLAB Function8 : MATLAB Function  TreatAsAtomicUnit=on
  Action : Outport
  wires:
  Gain1/1 -> MATLAB Function8/1(u)
  Gain4/1 -> MATLAB Function1/1(u)
  MATLAB Function8/1(y) -> Gain4/1
  observations/1 -> Gain1/1
  MATLAB Function1/1(y) -> Action/1

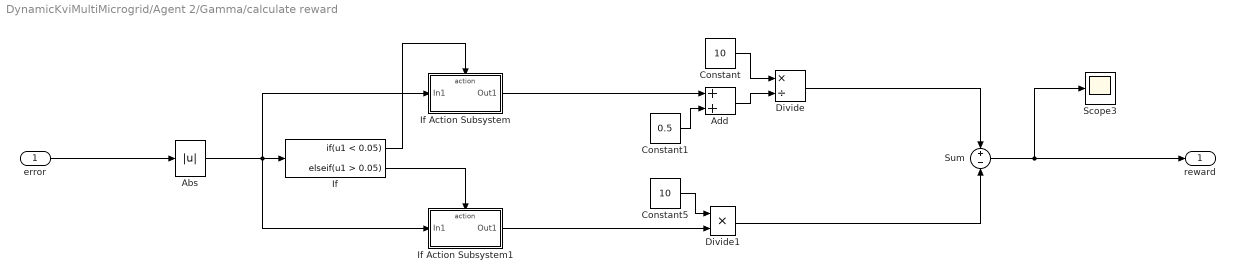
== system DynamicKviMultiMicrogrid/Agent 2/Gamma/calculate reward ==
  error : Inport
  Abs : Abs  SaturateOnIntegerOverflow=off
  Add : Sum
  Constant : Constant  Value=10
  Constant1 : Constant  Value=0.5  VectorParams1D=off
  Constant5 : Constant  Value=10  VectorParams1D=off
  Divide : Product  Inputs=*/
  Divide1 : Product  Inputs=**
  If : If  IfExpression=u1 < 0.05  ElseIfExpressions=u1 > 0.05  ShowElse=off
  If Action Subsystem : Subsystem  TreatAsAtomicUnit=on
  If Action Subsystem1 : Subsystem  TreatAsAtomicUnit=on
  Scope3 : Scope
  Sum : Sum  Inputs=+-  OutDataTypeStr=double
  reward : Outport  VectorParamsAs1DForOutWhenUnconnected=off
  wires:
  Constant/1 -> Divide/1
  Add/1 -> Divide/2
  Constant1/1 -> Add/2
  error/1 -> Abs/1
  Constant5/1 -> Divide1/1
  If Action Subsystem1/1(Out1) -> Divide1/2
  Divide/1 -> Sum/1
  If Action Subsystem/1(Out1) -> Add/1
  Sum/1 -> Scope3/1, reward/1
  If/2 -> If Action Subsystem1/Action
  If/1 -> If Action Subsystem/Action
  Abs/1 -> If/1, If Action Subsystem1/1(In1), If Action Subsystem/1(In1)
  Divide1/1 -> Sum/2

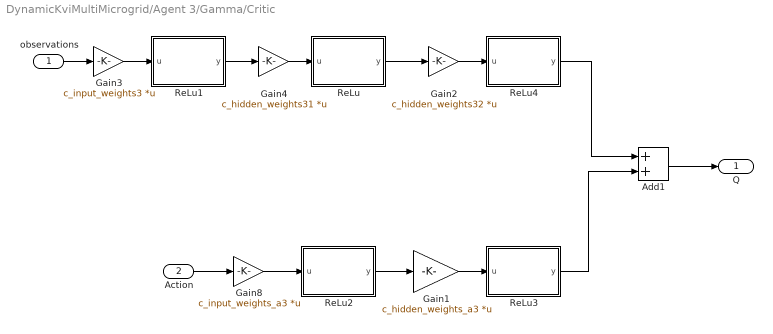
== system DynamicKviMultiMicrogrid/Agent 3/Gamma/Critic ==
  observations : Inport
  Action : Inport  Port=2
  Add1 : Sum
  Gain1 : Gain  Gain=c_hidden_weights_a3  Multiplication=Matrix(K*u)
  Gain2 : Gain  Gain=c_hidden_weights32  Multiplication=Matrix(K*u)
  Gain3 : Gain  Gain=c_input_weights3  Multiplication=Matrix(K*u)
  Gain4 : Gain  Gain=c_hidden_weights31  Multiplication=Matrix(K*u)
  Gain8 : Gain  Gain=c_input_weights_a3  Multiplication=Matrix(K*u)
  ReLu : MATLAB Function  TreatAsAtomicUnit=on
  ReLu1 : MATLAB Function  TreatAsAtomicUnit=on
  ReLu2 : MATLAB Function  TreatAsAtomicUnit=on
  ReLu3 : MATLAB Function  TreatAsAtomicUnit=on
  ReLu4 : MATLAB Function  TreatAsAtomicUnit=on
  Q : Outport
  wires:
  observations/1 -> Gain3/1
  Add1/1 -> Q/1
  Action/1 -> Gain8/1
  ReLu3/1(y) -> Add1/2
  Gain8/1 -> ReLu2/1(u)
  ReLu2/1(y) -> Gain1/1
  Gain1/1 -> ReLu3/1(u)
  Gain3/1 -> ReLu1/1(u)
  ReLu1/1(y) -> Gain4/1
  Gain4/1 -> ReLu/1(u)
  ReLu/1(y) -> Gain2/1
  Gain2/1 -> ReLu4/1(u)
  ReLu4/1(y) -> Add1/1

== system DynamicKviMultiMicrogrid/Agent 3/Gamma/NN Controller ==
  observations : Inport
  Gain1 : Gain  Gain=a_input_weights3(:,:)  Multiplication=Matrix(K*u)
  Gain4 : Gain  Gain=a_hidden_weights3(:,:)  Multiplication=Matrix(K*u)
  MATLAB Function1 : MATLAB Function  TreatAsAtomicUnit=on
  MATLAB Function8 : MATLAB Function  TreatAsAtomicUnit=on
  Action : Outport
  wires:
  Gain1/1 -> MATLAB Function8/1(u)
  Gain4/1 -> MATLAB Function1/1(u)
  MATLAB Function8/1(y) -> Gain4/1
  observations/1 -> Gain1/1
  MATLAB Function1/1(y) -> Action/1

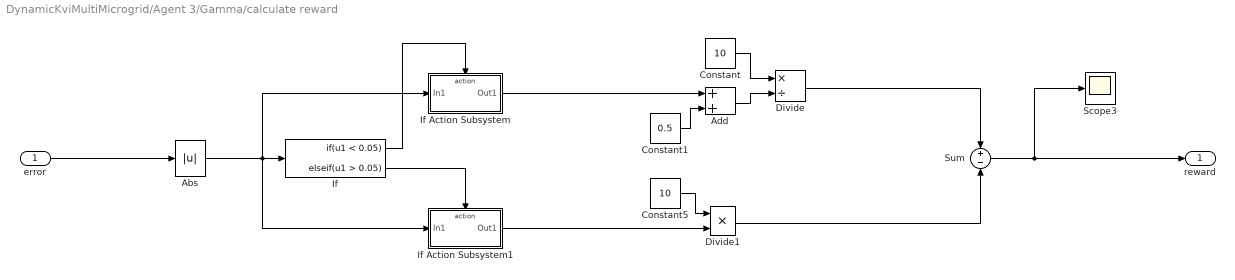
== system DynamicKviMultiMicrogrid/Agent 3/Gamma/calculate reward ==
  error : Inport
  Abs : Abs  SaturateOnIntegerOverflow=off
  Add : Sum
  Constant : Constant  Value=10
  Constant1 : Constant  Value=0.5  VectorParams1D=off
  Constant5 : Constant  Value=10  VectorParams1D=off
  Divide : Product  Inputs=*/
  Divide1 : Product  Inputs=**
  If : If  IfExpression=u1 < 0.05  ElseIfExpressions=u1 > 0.05  ShowElse=off
  If Action Subsystem : Subsystem  TreatAsAtomicUnit=on
  If Action Subsystem1 : Subsystem  TreatAsAtomicUnit=on
  Scope3 : Scope
  Sum : Sum  Inputs=+-  OutDataTypeStr=double
  reward : Outport  VectorParamsAs1DForOutWhenUnconnected=off
  wires:
  Constant/1 -> Divide/1
  Add/1 -> Divide/2
  Constant1/1 -> Add/2
  error/1 -> Abs/1
  Constant5/1 -> Divide1/1
  If Action Subsystem1/1(Out1) -> Divide1/2
  Divide/1 -> Sum/1
  If Action Subsystem/1(Out1) -> Add/1
  Sum/1 -> Scope3/1, reward/1
  If/2 -> If Action Subsystem1/Action
  If/1 -> If Action Subsystem/Action
  Abs/1 -> If/1, If Action Subsystem1/1(In1), If Action Subsystem/1(In1)
  Divide1/1 -> Sum/2

== system DynamicKviMultiMicrogrid/Agent 1/Gamma/calculate reward/If Action Subsystem ==
  In1 : Inport
  Action Port : ActionPort  ActionPortLabel=if(u1 < 0.05)
  Out1 : Outport
  wires:
  In1/1 -> Out1/1

== system DynamicKviMultiMicrogrid/Agent 1/Gamma/calculate reward/If Action Subsystem1 ==
  In1 : Inport
  Action Port : ActionPort  ActionPortLabel=elseif(u1 > 0.05)
  Out1 : Outport
  wires:
  In1/1 -> Out1/1

== system DynamicKviMultiMicrogrid/Agent 2/Gamma/calculate reward/If Action Subsystem ==
  In1 : Inport
  Action Port : ActionPort  ActionPortLabel=if(u1 < 0.05)
  Out1 : Outport
  wires:
  In1/1 -> Out1/1

== system DynamicKviMultiMicrogrid/Agent 2/Gamma/calculate reward/If Action Subsystem1 ==
  In1 : Inport
  Action Port : ActionPort  ActionPortLabel=elseif(u1 > 0.05)
  Out1 : Outport
  wires:
  In1/1 -> Out1/1

== system DynamicKviMultiMicrogrid/Agent 3/Gamma/calculate reward/If Action Subsystem ==
  In1 : Inport
  Action Port : ActionPort  ActionPortLabel=if(u1 < 0.05)
  Out1 : Outport
  wires:
  In1/1 -> Out1/1

== system DynamicKviMultiMicrogrid/Agent 3/Gamma/calculate reward/If Action Subsystem1 ==
  In1 : Inport
  Action Port : ActionPort  ActionPortLabel=elseif(u1 > 0.05)
  Out1 : Outport
  wires:
  In1/1 -> Out1/1

== matlab function DynamicKviMultiMicrogrid/Agent 2/Gamma/NN Controller/MATLAB Function1 ==
  data: u input; y output
function y = fcn(u)
y=ones(size(u));
for i=1:1
y(i)=(10/(1+exp(-abs(0.5*u(i))))-5);
end
end

== matlab function DynamicKviMultiMicrogrid/Agent 2/Gamma/NN Controller/MATLAB Function8 ==
  data: u input; y output
function y = fcn(u)
y=ones(size(u));
for i=1:3
y(i)=(10/(1+exp(-abs(0.5*u(i))))-5);
end
end

== matlab function DynamicKviMultiMicrogrid/Agent 2/Gamma/Critic/ReLu ==
  data: u input; y output
function y = fcn(u)
y=ones(size(u));
for i=1:100
 if u>0
    y(i)=u(i);
 else
    y(i)=u(i)*0.01;
 end
end

end

== matlab function DynamicKviMultiMicrogrid/Agent 2/Gamma/Critic/ReLu1 ==
  data: u input; y output
function y = fcn(u)
y=ones(size(u));
for i=1:1000
 if u>0
    y(i)=u(i);
 else
    y(i)=u(i)*0.01;
 end
end

end

== matlab function DynamicKviMultiMicrogrid/Agent 2/Gamma/Critic/ReLu2 ==
  data: u input; y output
function y = fcn(u)
y=ones(size(u));
for i=1:100
 if u>0
    y(i)=u(i);
 else
    y(i)=u(i)*0.01;
 end
end

end

== matlab function DynamicKviMultiMicrogrid/Agent 3/Gamma/Critic/ReLu1 ==
  data: u input; y output
function y = fcn(u)
y=ones(size(u));
for i=1:1000
 if u>0
    y(i)=u(i);
 else
    y(i)=u(i)*0.01;
 end
end

end

== matlab function DynamicKviMultiMicrogrid/Agent 2/Gamma/Critic/ReLu3 ==
  data: u input; y output
function y = fcn(u)
y=ones(size(u));
for i=1:1
 if u>0
    y(i)=u(i);
 else
    y(i)=u(i)*0.01;
 end
end

end

== matlab function DynamicKviMultiMicrogrid/Agent 2/Gamma/Critic/ReLu4 ==
  data: u input; y output
function y = fcn(u)
y=ones(size(u));
for i=1:1
 if u>0
    y(i)=u(i);
 else
    y(i)=u(i)*0.01;
 end
end

end

== matlab function DynamicKviMultiMicrogrid/Agent 3/Gamma/Critic/ReLu2 ==
  data: u input; y output
function y = fcn(u)
y=ones(size(u));
for i=1:100
 if u>0
    y(i)=u(i);
 else
    y(i)=u(i)*0.01;
 end
end

end

== matlab function DynamicKviMultiMicrogrid/Agent 3/Gamma/Critic/ReLu3 ==
  data: u input; y output
function y = fcn(u)
y=ones(size(u));
for i=1:1
 if u>0
    y(i)=u(i);
 else
    y(i)=u(i)*0.01;
 end
end

end

== matlab function DynamicKviMultiMicrogrid/Agent 3/Gamma/Critic/ReLu4 ==
  data: u input; y output
function y = fcn(u)
y=ones(size(u));
for i=1:1
 if u>0
    y(i)=u(i);
 else
    y(i)=u(i)*0.01;
 end
end

end

== matlab function DynamicKviMultiMicrogrid/Agent 3/Gamma/NN Controller/MATLAB Function1 ==
  data: u input; y output
function y = fcn(u)
y=ones(size(u));
for i=1:1
y(i)=(10/(1+exp(-abs(0.5*u(i))))-5);
end
end

== matlab function DynamicKviMultiMicrogrid/Agent 3/Gamma/NN Controller/MATLAB Function8 ==
  data: u input; y output
function y = fcn(u)
y=ones(size(u));
for i=1:3
y(i)=(10/(1+exp(-abs(0.5*u(i))))-5);
end
end

== matlab function DynamicKviMultiMicrogrid/Agent 1/Gamma/Critic/ReLu ==
  data: u input; y output
function y = fcn(u)
y=ones(size(u));
for i=1:100
 if u>0
    y(i)=u(i);
 else
    y(i)=u(i)*0.01;
 end
end

end

== matlab function DynamicKviMultiMicrogrid/Agent 1/Gamma/Critic/ReLu1 ==
  data: u input; y output
function y = fcn(u)
y=ones(size(u));
for i=1:1000
 if u>0
    y(i)=u(i);
 else
    y(i)=u(i)*0.01;
 end
end

end

== matlab function DynamicKviMultiMicrogrid/Agent 3/Gamma/Critic/ReLu ==
  data: u input; y output
function y = fcn(u)
y=ones(size(u));
for i=1:100
 if u>0
    y(i)=u(i);
 else
    y(i)=u(i)*0.01;
 end
end

end

== matlab function DynamicKviMultiMicrogrid/Agent 1/Gamma/Critic/ReLu2 ==
  data: u input; y output
function y = fcn(u)
y=ones(size(u));
for i=1:100
 if u>0
    y(i)=u(i);
 else
    y(i)=u(i)*0.01;
 end
end

end

== matlab function DynamicKviMultiMicrogrid/Agent 1/Gamma/Critic/ReLu3 ==
  data: u input; y output
function y = fcn(u)
y=ones(size(u));
for i=1:1
 if u>0
    y(i)=u(i);
 else
    y(i)=u(i)*0.01;
 end
end

end

== matlab function DynamicKviMultiMicrogrid/Agent 1/Gamma/Critic/ReLu4 ==
  data: u input; y output
function y = fcn(u)
y=ones(size(u));
for i=1:1
 if u>0
    y(i)=u(i);
 else
    y(i)=u(i)*0.01;
 end
end

end

== matlab function DynamicKviMultiMicrogrid/Agent 1/Gamma/NN Controller/MATLAB Function1 ==
  data: u input; y output
function y = fcn(u)
y=ones(size(u));
for i=1:1
y(i)=(10/(1+exp(-abs(0.5*u(i))))-5);
end
end

== matlab function DynamicKviMultiMicrogrid/Agent 1/Gamma/NN Controller/MATLAB Function8 ==
  data: u input; y output
function y = fcn(u)
y=ones(size(u));
for i=1:3
y(i)=(10/(1+exp(-abs(0.5*u(i))))-5);
end
end
